simulink model "stockBot"  (R2021a)
settings: Solver=VariableStepAuto  StartTime=0.0  StopTime=10.0  RelTol=1e-3
libraries: rllib x1
settings Model: Creator=Mitch  LastModifiedBy=Mitch

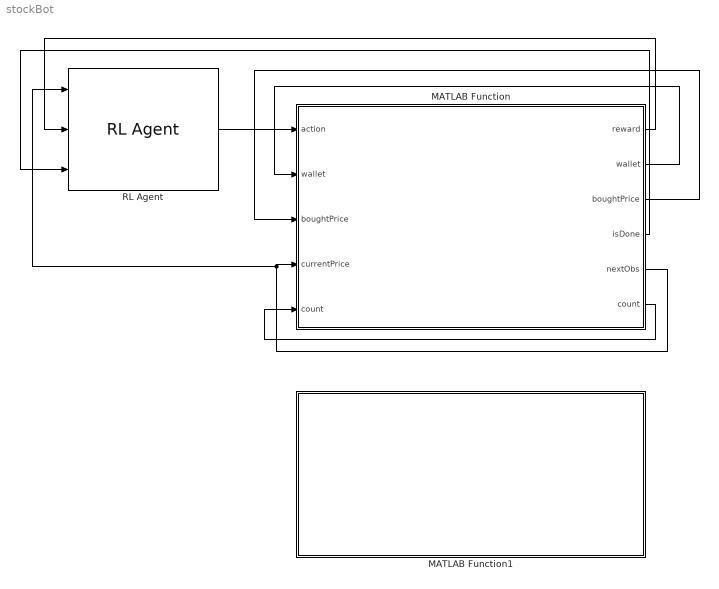
== system stockBot ==
  MATLAB Function : MATLAB Function  InitFcn=|  TreatAsAtomicUnit=on
      | wallet = 500;
      | boughtPrice = 0;
      | count = 0;
  MATLAB Function1 : MATLAB Function  TreatAsAtomicUnit=on
  RL Agent : rllib/RL Agent  Agent=Tony  ExternalActionAsInput=off  ProvideCumRwd=off  TreatAsDirectFeedthrough=on
  wires:
  RL Agent/1 -> MATLAB Function/1(action)
  MATLAB Function/2(wallet) -> MATLAB Function/2("wallet ")
  MATLAB Function/1(reward) -> RL Agent/2
  MATLAB Function/3(boughtPrice) -> MATLAB Function/3("boughtPrice ")
  MATLAB Function/4(isDone) -> RL Agent/3
  MATLAB Function/5(nextObs) -> RL Agent/1, MATLAB Function/4(currentPrice)
  MATLAB Function/6(count) -> MATLAB Function/5("count ")

== matlab function stockBot/MATLAB Function1 ==
function myResetFunction

y = u;

== matlab function stockBot/MATLAB Function ==
  data: action input; wallet input; boughtPrice input; reward output; currentPrice input; wallet output; boughtPrice output; isDone output; nextObs output; count output; count input
function [reward, wallet, boughtPrice, isDone, nextObs, count] = buyOrSell(action, wallet, boughtPrice, currentPrice, count)
load("dataset\oneLine.mat");

count = count + 1;
nextObs = data(count);

if((action <= -0.5) && (boughtPrice ~= 0))          %Sell
    reward = boughtPrice - currentPrice;
    wallet = wallet + currentPrice;
    
elseif((action >= 0.5) && (wallet >= currentPrice)) %Buy
    boughtPrice = currentPrice;
    wallet = wallet - currentPrice;
    reward = - currentPrice;
    
else                                                %Hold
    reward = 0;
end
    
if(wallet >= 1000)
    isDone = 1;
else
    isDone = 0;
end
    


end
